simulink model "testing"  (R2020a)
settings: Solver=VariableStepAuto  StartTime=0.0  StopTime=20  RelTol=1e-3
libraries: sps_avr x21, powerlib x17, powerlib_meascontrol x6, spsDieselMotorModel x3
settings Model: Creator=assem  LastModifiedBy=assem

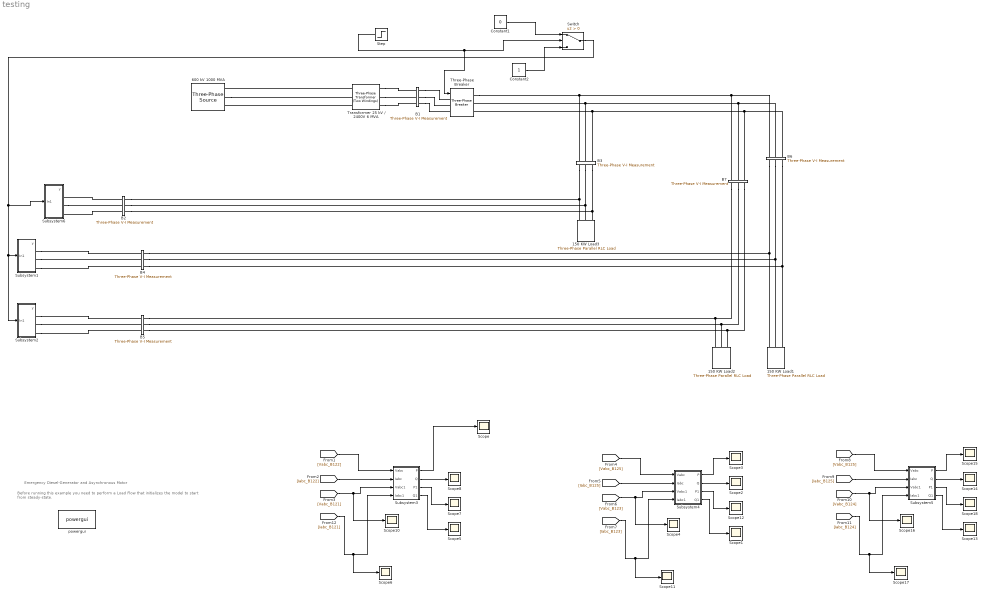
== system testing ==
  note: Emergency Diesel-Generator and Asynchronous Motor
  note: Before running this example you need to perform a Load Flow that
      | initializes the model to start from steady-state.
  150 KW Load1 : powerlib/Elements/Three-Phase Parallel RLC Load  LConnTagsString=A|B|C  Configuration=Y (grounded)  NominalVoltage=2400  Vabc=[1e3 1e3 1e3]  Vabcp=[1e3 1e3 1e3]  NominalFrequency=60  UnbalancedPower=off  ActivePower=.15e+006  InductivePower=0  CapacitivePower=0  Pabc=[10e3 9e3 11e3]  QLabc=[100 90 110]  QCabc=[100 90 110]  Pabcp=[10e3 9e3 11e3]  QLabcp=[100 90 110]  QCabcp=[100 90 110]  Measurements=None  LoadType=constant Z
      settings: SourceProductBaseCode=MT,PS
  150 KW Load2 : powerlib/Elements/Three-Phase Parallel RLC Load  LConnTagsString=A|B|C  Configuration=Y (grounded)  NominalVoltage=2400  Vabc=[1e3 1e3 1e3]  Vabcp=[1e3 1e3 1e3]  NominalFrequency=60  UnbalancedPower=off  ActivePower=.15e+006  InductivePower=0  CapacitivePower=0  Pabc=[10e3 9e3 11e3]  QLabc=[100 90 110]  QCabc=[100 90 110]  Pabcp=[10e3 9e3 11e3]  QLabcp=[100 90 110]  QCabcp=[100 90 110]  Measurements=None  LoadType=constant Z
      settings: SourceProductBaseCode=MT,PS
  150 KW Load3 : powerlib/Elements/Three-Phase Parallel RLC Load  LConnTagsString=A|B|C  Configuration=Y (grounded)  NominalVoltage=2400  Vabc=[1e3 1e3 1e3]  Vabcp=[1e3 1e3 1e3]  NominalFrequency=60  UnbalancedPower=off  ActivePower=.2e+006  InductivePower=0  CapacitivePower=0  Pabc=[10e3 9e3 11e3]  QLabc=[100 90 110]  QCabc=[100 90 110]  Pabcp=[10e3 9e3 11e3]  QLabcp=[100 90 110]  QCabcp=[100 90 110]  Measurements=None  LoadType=constant Z
      settings: SourceProductBaseCode=MT,PS
  600 kV 1000 MVA : powerlib/Electrical Sources/Three-Phase Source  InternalConnection=Yg  VoltagePhases=off  Voltage=(13800)*1  PhaseAngle=0.071468  Voltage_phases=[25e3 25e3 25e3]/sqrt(3)  PhaseAngles_phases=[0 -120 +120]  Frequency=60  NonIdealSource=on  SpecifyImpedance=on  Resistance=25^2/1000/10  Inductance=25^2/1000/377  ShortCircuitLevel=1000e6  BaseVoltage=13.8e3  XRratio=7  BusType=swing  Pref=0  Qref=0  Prefabc=[10e3, 10e3, 10e3]  Qrefabc=[0, 0, 0]  Qmin=-Inf  Qmax=Inf
      settings: SourceProductBaseCode=MT,PS
  B1 : powerlib/Measurements/Three-Phase V-I Measurement  VoltageMeasurement=phase-to-ground  SetLabelV=on  LabelV=Vabc_B120  Vpu=off  VpuLL=off  CurrentMeasurement=yes  SetLabelI=on  LabelI=Iabc_B120  Ipu=off  Pbase=100e6  Vbase=120e3  OutputType=Complex  PhasorSimulation=on  PSBequivalent=0
      settings: SourceProductBaseCode=MT,PS
  B2 : powerlib/Measurements/Three-Phase V-I Measurement  VoltageMeasurement=phase-to-ground  SetLabelV=on  LabelV=Vabc_B121  Vpu=off  VpuLL=off  CurrentMeasurement=yes  SetLabelI=on  LabelI=Iabc_B121  Ipu=off  Pbase=100e6  Vbase=120e3  OutputType=Complex  PhasorSimulation=on  PSBequivalent=0
      settings: SourceProductBaseCode=MT,PS
  B3 : powerlib/Measurements/Three-Phase V-I Measurement  VoltageMeasurement=phase-to-ground  SetLabelV=on  LabelV=Vabc_B122  Vpu=off  VpuLL=off  CurrentMeasurement=yes  SetLabelI=on  LabelI=Iabc_B122  Ipu=off  Pbase=100e6  Vbase=120e3  OutputType=Complex  PhasorSimulation=on  PSBequivalent=0
      settings: SourceProductBaseCode=MT,PS
  B4 : powerlib/Measurements/Three-Phase V-I Measurement  VoltageMeasurement=phase-to-ground  SetLabelV=on  LabelV=Vabc_B123  Vpu=off  VpuLL=off  CurrentMeasurement=yes  SetLabelI=on  LabelI=Iabc_B123  Ipu=off  Pbase=100e6  Vbase=120e3  OutputType=Complex  PhasorSimulation=on  PSBequivalent=0
      settings: SourceProductBaseCode=MT,PS
  B5 : powerlib/Measurements/Three-Phase V-I Measurement  VoltageMeasurement=phase-to-ground  SetLabelV=on  LabelV=Vabc_B124  Vpu=off  VpuLL=off  CurrentMeasurement=yes  SetLabelI=on  LabelI=Iabc_B124  Ipu=off  Pbase=100e6  Vbase=120e3  OutputType=Complex  PhasorSimulation=on  PSBequivalent=0
      settings: SourceProductBaseCode=MT,PS
  B6 : powerlib/Measurements/Three-Phase V-I Measurement  VoltageMeasurement=phase-to-ground  SetLabelV=on  LabelV=Vabc_B125  Vpu=off  VpuLL=off  CurrentMeasurement=yes  SetLabelI=on  LabelI=Iabc_B125  Ipu=off  Pbase=100e6  Vbase=120e3  OutputType=Complex  PhasorSimulation=on  PSBequivalent=0
      settings: SourceProductBaseCode=MT,PS
  B7 : powerlib/Measurements/Three-Phase V-I Measurement  VoltageMeasurement=phase-to-ground  SetLabelV=on  LabelV=Vabc_B126  Vpu=off  VpuLL=off  CurrentMeasurement=yes  SetLabelI=on  LabelI=Iabc_B126  Ipu=off  Pbase=100e6  Vbase=120e3  OutputType=Complex  PhasorSimulation=on  PSBequivalent=0
      settings: SourceProductBaseCode=MT,PS
  Constant1 : Constant  Value=0  SampleTime=1
  Constant2 : Constant  SampleTime=1
  Scope{,1..8,10..18} (18 alike) : Scope
  Step : Step  Time=4  Before=1  After=0  SampleTime=0
  Subsystem1 : Subsystem
  Subsystem2 : Subsystem
  Subsystem3 : Subsystem
  Subsystem4 : Subsystem
  Subsystem5 : Subsystem
  Subsystem6 : Subsystem
  Switch : Switch  Criteria=u2 > Threshold
  Three-Phase Breaker : powerlib/Elements/Three-Phase Breaker  InitialState=closed  SwitchA=on  SwitchB=on  SwitchC=on  SwitchTimes="[1/60  5/60]"  External=on  BreakerResistance=0.01  SnubberResistance=1e6  SnubberCapacitance=inf  Measurements=None
  Transformer 25 kV / 2400V 6 MVA : powerlib/Elements/Three-Phase Transformer (Two Windings)  Winding1Connection=Yg  Winding2Connection=Yg  CoreType=Three single-phase transformers  SetSaturation=off  Hysteresis=off  DataFile='hysteresis'  SetInitialFlux=off  Measurements=None  UNITS=pu  NominalPower=[ 5e6 , 60 ]  Winding1=[13.8e3 0.0015 0.03]  Winding2=[2.4e3 0.0015 0.03]  Rm=200  Lm=200  L0=3.7357e-08  Saturation=[0 0;0.005 1.2;1 1.4]  InitialFluxes=[0.022525 -0.022525 0.019709]  BreakLoop=off  DiscreteSolver=Trapezoidal iterative  DataType=off  TransfoNumber=0
      settings: SourceProductBaseCode=MT,PS
  powergui : powerlib/powergui  Priority=2  SimulationMode=Continuous  SampleTime=50e-6  frequency=60  Iterations=50  frequencyindice=60  Pbase=1e6  ErrMax=0.0001  UnitsV=kV  UnitsW=MW  buscounter=0  FunctionMessages=off  echomessages=off  EnableUseOfTLC=off  CurrentSourceSwitches=off  DisableSnubberDevices=on  DisableRonSwitches=off  DisableVfSwitches=off  DisplayEquations=off  AutomaticDiscreteSolvers=off  SolverType=Tustin  Interpol=off  ExternalGateDelay=off  methode=off  Ts=0  x0status=blocks  SPID=on  SwTol=0  HookPort=off  NonlinearTolerance=1e-4  nMaxIteration=100  ContinueOnMaxIteration=off  RestoreLinks=warning  ResistiveCurrentMeasurement=off  Frange=logspace(0,3,50)  Ylog=off  Xlog=off  ShowGrid=off  save=off  variable=ZData  structure=0  ZoomFFT=on  StartTime=0.0  cycles=2  DisplayStyle=off  fundamental=60  FreqAxis=off  MaxFrequency=1000  frequencyindicesteady=1  RmsSteady=1  display=off
  wires:
  Step/1 -> Three-Phase Breaker/1, Switch/2
  Constant2/1 -> Switch/3
  Constant1/1 -> Switch/1
  Switch/1 -> Subsystem6/1(In1), Subsystem2/1(In1), Subsystem1/1(In1)
  [Vabc_B123] -> Subsystem4/3(Vabc1), Scope4/1
  [Iabc_B123] -> Subsystem4/4(Iabc1), Scope11/1
  Subsystem4/4(Q1) -> Scope1/1
  Subsystem4/1(P) -> Scope3/1
  [Vabc_B125] -> Subsystem4/1(Vabc)
  [Iabc_B125] -> Subsystem4/2(Iabc)
  Subsystem4/2(Q) -> Scope2/1
  Subsystem4/3(P1) -> Scope12/1
  [Vabc_B124] -> Subsystem5/3(Vabc1), Scope16/1
  [Iabc_B124] -> Subsystem5/4(Iabc1), Scope17/1
  Subsystem5/4(Q1) -> Scope13/1
  Subsystem5/1(P) -> Scope15/1
  [Vabc_B125] -> Subsystem5/1(Vabc)
  [Iabc_B125] -> Subsystem5/2(Iabc)
  Subsystem5/2(Q) -> Scope14/1
  Subsystem5/3(P1) -> Scope18/1
  Subsystem3/2(Q) -> Scope8/1
  Subsystem3/3(P1) -> Scope7/1
  [Iabc_B122] -> Subsystem3/2(Iabc)
  [Vabc_B122] -> Subsystem3/1(Vabc)
  [Iabc_B121] -> Subsystem3/4(Iabc1), Scope6/1
  [Vabc_B121] -> Subsystem3/3(Vabc1), Scope10/1
  Subsystem3/4(Q1) -> Scope5/1
  Subsystem3/1(P) -> Scope/1
  connections:
  B1/RConn3 -- Three-Phase Breaker/LConn3
  600 kV 1000 MVA/RConn2 -- Transformer 25 kV / 2400V 6 MVA/LConn2
  Transformer 25 kV / 2400V 6 MVA/RConn1 -- B1/LConn1
  Three-Phase Breaker/RConn1 -- B3/LConn3 -- B7/LConn3 -- B6/RConn3
  B1/RConn2 -- Three-Phase Breaker/LConn2
  Transformer 25 kV / 2400V 6 MVA/RConn2 -- B1/LConn2
  B1/RConn1 -- Three-Phase Breaker/LConn1
  Transformer 25 kV / 2400V 6 MVA/LConn3 -- 600 kV 1000 MVA/RConn3
  Transformer 25 kV / 2400V 6 MVA/LConn1 -- 600 kV 1000 MVA/RConn1
  B6/RConn1 -- B3/LConn1 -- Three-Phase Breaker/RConn3 -- B7/LConn1
  Transformer 25 kV / 2400V 6 MVA/RConn3 -- B1/LConn3
  B6/RConn2 -- B3/LConn2 -- Three-Phase Breaker/RConn2 -- B7/LConn2
  Subsystem1/RConn1 -- B4/LConn1
  Subsystem1/RConn2 -- B4/LConn2
  Subsystem1/RConn3 -- B4/LConn3
  Subsystem2/RConn1 -- B5/LConn1
  Subsystem2/RConn2 -- B5/LConn2
  Subsystem2/RConn3 -- B5/LConn3
  B4/RConn3 -- B6/LConn1 -- 150 KW Load1/LConn3
  B4/RConn2 -- B6/LConn2 -- 150 KW Load1/LConn2
  B4/RConn1 -- B6/LConn3 -- 150 KW Load1/LConn1
  B5/RConn3 -- B7/RConn1 -- 150 KW Load2/LConn3
  B5/RConn2 -- B7/RConn2 -- 150 KW Load2/LConn2
  B5/RConn1 -- B7/RConn3 -- 150 KW Load2/LConn1
  B2/LConn1 -- Subsystem6/RConn1
  Subsystem6/RConn2 -- B2/LConn2
  B2/LConn3 -- Subsystem6/RConn3
  B3/RConn1 -- B2/RConn3 -- 150 KW Load3/LConn3
  B3/RConn2 -- B2/RConn2 -- 150 KW Load3/LConn2
  B3/RConn3 -- B2/RConn1 -- 150 KW Load3/LConn1

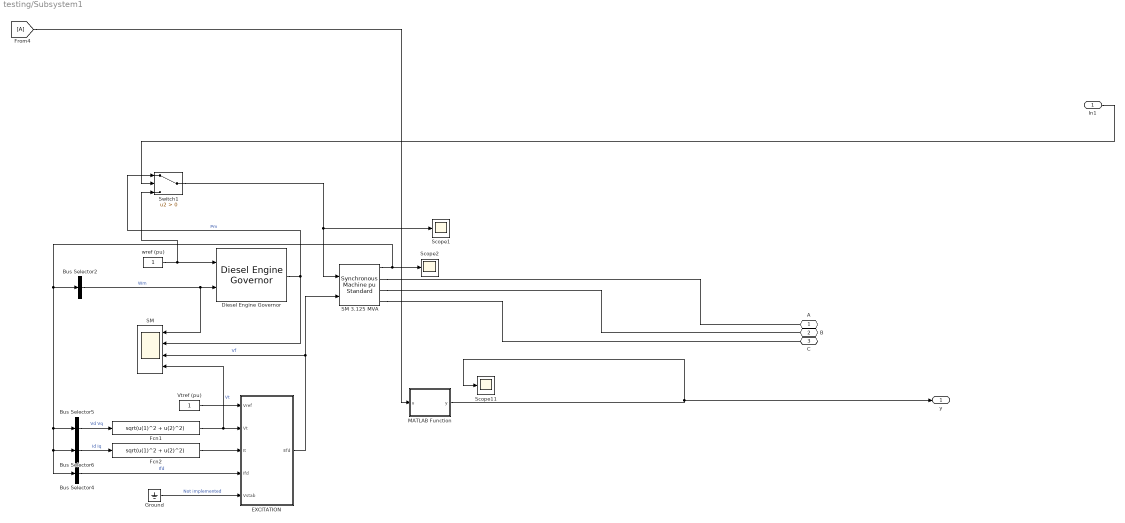
== system testing/Subsystem1 ==
  In1 : Inport
  Bus Selector2 : BusSelector  OutputSignals="Mechanical.Rotor speed  wm  (pu)"  OutputAsBus=on
  Bus Selector4 : BusSelector  OutputSignals="dq0 components.Field current  ifd (pu)"  OutputAsBus=on
  Bus Selector5 : BusSelector  OutputSignals="dq0 components.Stator voltage  vd (pu),dq0 components.Stator voltage  vq (pu)"  OutputAsBus=on
  Bus Selector6 : BusSelector  OutputSignals="dq0 components.Stator current  id (pu),dq0 components.Stator current  iq (pu)"  OutputAsBus=on
  Diesel Engine Governor : spsDieselMotorModel/Diesel Engine Governor  K=40  Tr=[0.01 0.02 0.2]  Ta=[0.25 0.009 0.0384]  Tlim=[0 1.1]  Td=0.024  Pm0=0
      settings: SourceProductBaseCode=MT,PS
  EXCITATION : Subsystem  Variant=on  VariantControlMode=Label  LabelModeActiveChoice=Variant1
      settings: AttributesFormatString=%<BlockChoice>
  Fcn1 : Fcn  Expr=sqrt(u(1)^2 + u(2)^2)
  Fcn2 : Fcn  Expr=sqrt(u(1)^2 + u(2)^2)
  Ground : Ground
  MATLAB Function : MATLAB Function  TreatAsAtomicUnit=on
  SM : Scope  NumInputPorts=4
  SM 3.125 MVA : powerlib/Machines/Synchronous Machine pu Standard  PresetModel=No  MechanicalLoad=Mechanical power Pm  ShowDetailedParameters=on  RotorType=Salient-pole  Units=per unit standard parameters  MeasurementBus=off  NominalParameters="[ .7e6  2400  60]"  Reactances1=[ 31 32 33 34 35 36 37 ]  Reactances2=[ 1.56, 0.296, 0.177, 1.06, 0.177, 0.052 ]  dAxisTimeConstants=Short-circuit  qAxisTimeConstants=Open-circuit  TimeConstants1=[]  TimeConstants2=[]  TimeConstants3=[]  TimeConstants4=[]  TimeConstants5=[ 3.7, 0.05, 0.05 ]  TimeConstants6=[ 8.0, 0.03, 0.3371, 0.0295 ]  TimeConstants7=[0.024 0.006 0.006]  TimeConstants8=[]  StatorResistance=0.0036  Mechanical="[ 1.07  0 2]"  PolePairs=2  InitialConditions=[0 0 0 0 0 0 0 0 1]  SetSaturation=off  Saturation=[0.211 0.418 1.0 1.25 1.72 3.35 ;0.25 0.50 1.0 1.1 1.2 1.4]  LoadFlowParameters=[1 0 0 0]  TsPowergui=0  TsBlock=-1  IterativeModel=Trapezoidal non iterative  IterativeDiscreteModel=Trapezoidal non iterative  BusType=swing  Pref=0  Qref=0  Qmin=-Inf  Qmax=Inf  PLF=0  QLF=0
      settings: AttributesFormatString=\n\n  SourceProductBaseCode=MT,PS
  Scope1 : Scope
  Scope11 : Scope
  Scope2 : Scope
  Switch1 : Switch  Criteria=u2 > Threshold
  "Vtref (pu) " : Constant
  wref (pu) : Constant
  A : PMIOPort  Side=Right
  B : PMIOPort  Port=2  Side=Right
  C : PMIOPort  Port=3  Side=Right
  y : Outport
  wires:
  Switch1/1 -> SM 3.125 MVA/1, Scope1/1
  In1/1 -> Switch1/2
  EXCITATION/1(Efd) -> SM/3, SM 3.125 MVA/2  "Vf"
  wref (pu)/1 -> Switch1/3, Diesel Engine Governor/1
  Bus Selector2/1 -> Diesel Engine Governor/2, SM/1  "Wm"
  "Vtref (pu) "/1 -> EXCITATION/1(Vref)
  Ground/1 -> EXCITATION/5(Vstab)  "Not implemented"
  Fcn2/1 -> EXCITATION/3(It)
  [A] -> MATLAB Function/1(u)
  SM 3.125 MVA/1 -> Bus Selector2/1, Bus Selector5/1, Bus Selector6/1, Bus Selector4/1, Scope2/1
  Bus Selector5/1 -> Fcn1/1  "Vd Vq"
  Fcn1/1 -> SM/4, EXCITATION/2(Vt)  "Vt"
  Bus Selector6/1 -> Fcn2/1  "Id Iq"
  Diesel Engine Governor/1 -> Switch1/1, SM/2  "Pm"
  Bus Selector4/1 -> EXCITATION/4(Ifd)  "Ifd"
  MATLAB Function/1(y) -> y/1, Scope11/1
  connections:
  SM 3.125 MVA/RConn3 -- C/RConn1
  SM 3.125 MVA/RConn1 -- A/RConn1
  SM 3.125 MVA/RConn2 -- B/RConn1

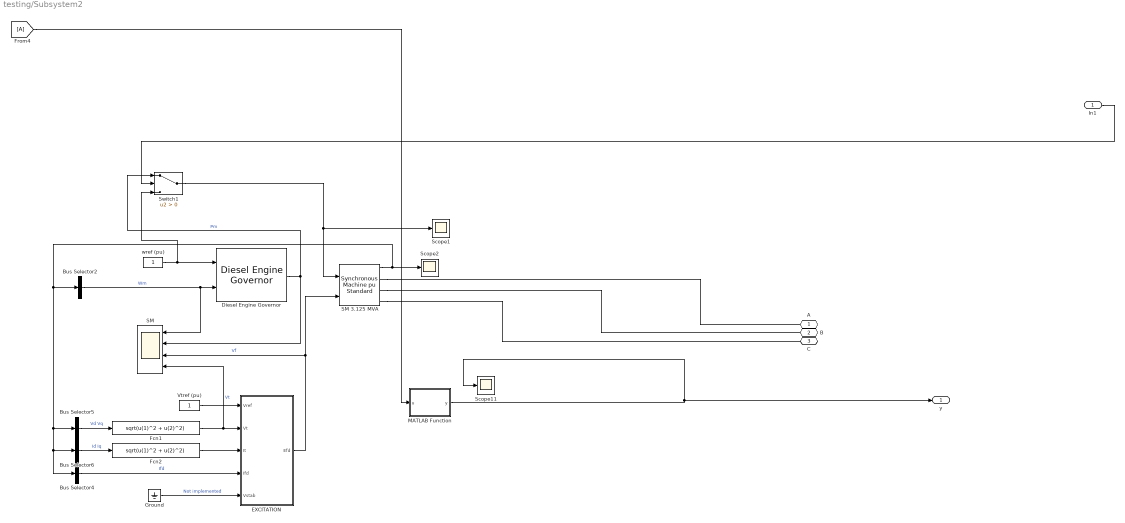
== system testing/Subsystem2 ==
  In1 : Inport
  Bus Selector2 : BusSelector  OutputSignals="Mechanical.Rotor speed  wm  (pu)"  OutputAsBus=on
  Bus Selector4 : BusSelector  OutputSignals="dq0 components.Field current  ifd (pu)"  OutputAsBus=on
  Bus Selector5 : BusSelector  OutputSignals="dq0 components.Stator voltage  vd (pu),dq0 components.Stator voltage  vq (pu)"  OutputAsBus=on
  Bus Selector6 : BusSelector  OutputSignals="dq0 components.Stator current  id (pu),dq0 components.Stator current  iq (pu)"  OutputAsBus=on
  Diesel Engine Governor : spsDieselMotorModel/Diesel Engine Governor  K=40  Tr=[0.01 0.02 0.2]  Ta=[0.25 0.009 0.0384]  Tlim=[0 1.1]  Td=0.024  Pm0=0
      settings: SourceProductBaseCode=MT,PS
  EXCITATION : Subsystem  Variant=on  VariantControlMode=Label  LabelModeActiveChoice=Variant1
      settings: AttributesFormatString=%<BlockChoice>
  Fcn1 : Fcn  Expr=sqrt(u(1)^2 + u(2)^2)
  Fcn2 : Fcn  Expr=sqrt(u(1)^2 + u(2)^2)
  Ground : Ground
  MATLAB Function : MATLAB Function  TreatAsAtomicUnit=on
  SM : Scope  NumInputPorts=4
  SM 3.125 MVA : powerlib/Machines/Synchronous Machine pu Standard  PresetModel=No  MechanicalLoad=Mechanical power Pm  ShowDetailedParameters=on  RotorType=Salient-pole  Units=per unit standard parameters  MeasurementBus=off  NominalParameters="[ .7e6  2400  60]"  Reactances1=[ 31 32 33 34 35 36 37 ]  Reactances2=[ 1.56, 0.296, 0.177, 1.06, 0.177, 0.052 ]  dAxisTimeConstants=Short-circuit  qAxisTimeConstants=Open-circuit  TimeConstants1=[]  TimeConstants2=[]  TimeConstants3=[]  TimeConstants4=[]  TimeConstants5=[ 3.7, 0.05, 0.05 ]  TimeConstants6=[ 8.0, 0.03, 0.3371, 0.0295 ]  TimeConstants7=[0.024 0.006 0.006]  TimeConstants8=[]  StatorResistance=0.0036  Mechanical="[ 1.07  0 2]"  PolePairs=2  InitialConditions=[0 0 0 0 0 0 0 0 1]  SetSaturation=off  Saturation=[0.211 0.418 1.0 1.25 1.72 3.35 ;0.25 0.50 1.0 1.1 1.2 1.4]  LoadFlowParameters=[1 0 0 0]  TsPowergui=0  TsBlock=-1  IterativeModel=Trapezoidal non iterative  IterativeDiscreteModel=Trapezoidal non iterative  BusType=swing  Pref=0  Qref=0  Qmin=-Inf  Qmax=Inf  PLF=0  QLF=0
      settings: AttributesFormatString=\n\n  SourceProductBaseCode=MT,PS
  Scope1 : Scope
  Scope11 : Scope
  Scope2 : Scope
  Switch1 : Switch  Criteria=u2 > Threshold
  "Vtref (pu) " : Constant
  wref (pu) : Constant
  A : PMIOPort  Side=Right
  B : PMIOPort  Port=2  Side=Right
  C : PMIOPort  Port=3  Side=Right
  y : Outport
  wires:
  Switch1/1 -> SM 3.125 MVA/1, Scope1/1
  In1/1 -> Switch1/2
  EXCITATION/1(Efd) -> SM/3, SM 3.125 MVA/2  "Vf"
  wref (pu)/1 -> Switch1/3, Diesel Engine Governor/1
  Bus Selector2/1 -> Diesel Engine Governor/2, SM/1  "Wm"
  "Vtref (pu) "/1 -> EXCITATION/1(Vref)
  Ground/1 -> EXCITATION/5(Vstab)  "Not implemented"
  Fcn2/1 -> EXCITATION/3(It)
  [A] -> MATLAB Function/1(u)
  SM 3.125 MVA/1 -> Bus Selector2/1, Bus Selector5/1, Bus Selector6/1, Bus Selector4/1, Scope2/1
  Bus Selector5/1 -> Fcn1/1  "Vd Vq"
  Fcn1/1 -> SM/4, EXCITATION/2(Vt)  "Vt"
  Bus Selector6/1 -> Fcn2/1  "Id Iq"
  Diesel Engine Governor/1 -> Switch1/1, SM/2  "Pm"
  Bus Selector4/1 -> EXCITATION/4(Ifd)  "Ifd"
  MATLAB Function/1(y) -> y/1, Scope11/1
  connections:
  SM 3.125 MVA/RConn3 -- C/RConn1
  SM 3.125 MVA/RConn1 -- A/RConn1
  SM 3.125 MVA/RConn2 -- B/RConn1

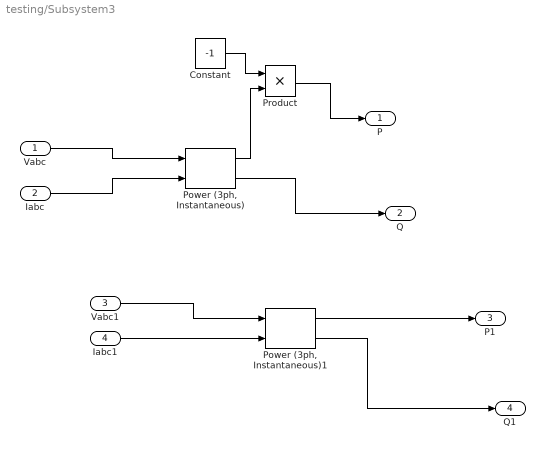
== system testing/Subsystem3 ==
  Vabc : Inport
  Iabc : Inport  Port=2
  Vabc1 : Inport  Port=3
  Iabc1 : Inport  Port=4
  Constant : Constant  Value=-1
  "Power (3ph, Instantaneous)" : powerlib_meascontrol/Measurements/Power (3ph, Instantaneous)
  "Power (3ph, Instantaneous)1" : powerlib_meascontrol/Measurements/Power (3ph, Instantaneous)
  Product : Product
  P : Outport
  Q : Outport  Port=2
  P1 : Outport  Port=3
  Q1 : Outport  Port=4
  wires:
  "Power (3ph, Instantaneous)1"/2 -> Q1/1
  Iabc/1 -> "Power (3ph, Instantaneous)"/2
  "Power (3ph, Instantaneous)1"/1 -> P1/1
  Iabc1/1 -> "Power (3ph, Instantaneous)1"/2
  "Power (3ph, Instantaneous)"/2 -> Q/1
  Vabc1/1 -> "Power (3ph, Instantaneous)1"/1
  Vabc/1 -> "Power (3ph, Instantaneous)"/1
  "Power (3ph, Instantaneous)"/1 -> Product/2
  Constant/1 -> Product/1
  Product/1 -> P/1

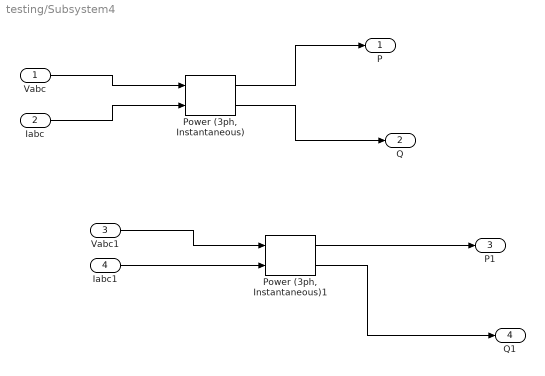
== system testing/Subsystem4 ==
  Vabc : Inport
  Iabc : Inport  Port=2
  Vabc1 : Inport  Port=3
  Iabc1 : Inport  Port=4
  "Power (3ph, Instantaneous)" : powerlib_meascontrol/Measurements/Power (3ph, Instantaneous)
  "Power (3ph, Instantaneous)1" : powerlib_meascontrol/Measurements/Power (3ph, Instantaneous)
  P : Outport
  Q : Outport  Port=2
  P1 : Outport  Port=3
  Q1 : Outport  Port=4
  wires:
  "Power (3ph, Instantaneous)1"/2 -> Q1/1
  "Power (3ph, Instantaneous)"/1 -> P/1
  Iabc/1 -> "Power (3ph, Instantaneous)"/2
  "Power (3ph, Instantaneous)1"/1 -> P1/1
  Iabc1/1 -> "Power (3ph, Instantaneous)1"/2
  "Power (3ph, Instantaneous)"/2 -> Q/1
  Vabc1/1 -> "Power (3ph, Instantaneous)1"/1
  Vabc/1 -> "Power (3ph, Instantaneous)"/1

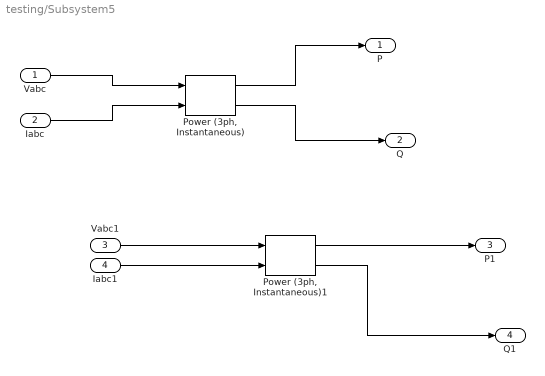
== system testing/Subsystem5 ==
  Vabc : Inport
  Iabc : Inport  Port=2
  Vabc1 : Inport  Port=3
  Iabc1 : Inport  Port=4
  "Power (3ph, Instantaneous)" : powerlib_meascontrol/Measurements/Power (3ph, Instantaneous)
  "Power (3ph, Instantaneous)1" : powerlib_meascontrol/Measurements/Power (3ph, Instantaneous)
  P : Outport
  Q : Outport  Port=2
  P1 : Outport  Port=3
  Q1 : Outport  Port=4
  wires:
  "Power (3ph, Instantaneous)1"/2 -> Q1/1
  "Power (3ph, Instantaneous)"/1 -> P/1
  Iabc/1 -> "Power (3ph, Instantaneous)"/2
  "Power (3ph, Instantaneous)1"/1 -> P1/1
  Iabc1/1 -> "Power (3ph, Instantaneous)1"/2
  "Power (3ph, Instantaneous)"/2 -> Q/1
  Vabc1/1 -> "Power (3ph, Instantaneous)1"/1
  Vabc/1 -> "Power (3ph, Instantaneous)"/1

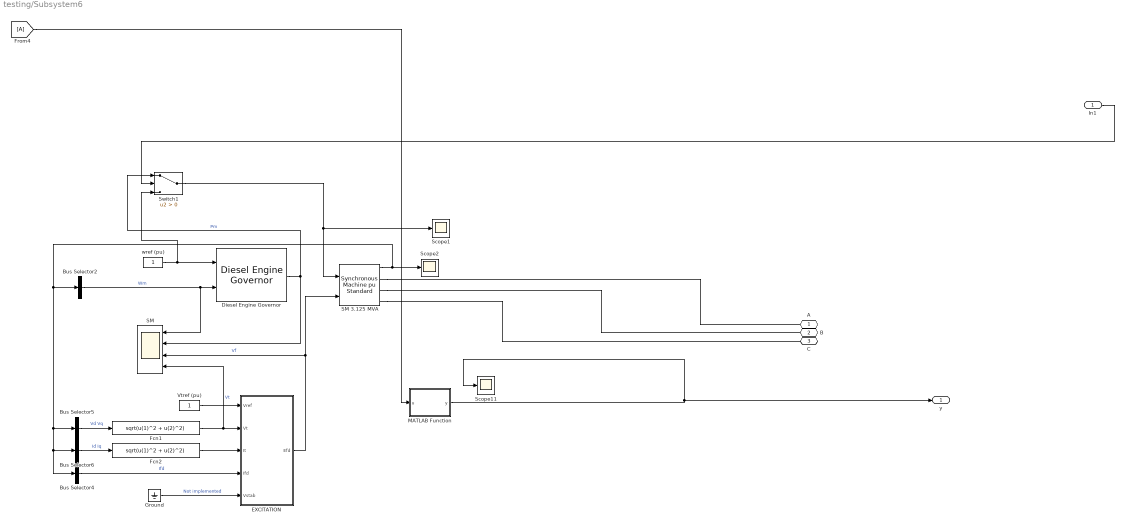
== system testing/Subsystem6 ==
  In1 : Inport
  Bus Selector2 : BusSelector  OutputSignals="Mechanical.Rotor speed  wm  (pu)"  OutputAsBus=on
  Bus Selector4 : BusSelector  OutputSignals="dq0 components.Field current  ifd (pu)"  OutputAsBus=on
  Bus Selector5 : BusSelector  OutputSignals="dq0 components.Stator voltage  vd (pu),dq0 components.Stator voltage  vq (pu)"  OutputAsBus=on
  Bus Selector6 : BusSelector  OutputSignals="dq0 components.Stator current  id (pu),dq0 components.Stator current  iq (pu)"  OutputAsBus=on
  Diesel Engine Governor : spsDieselMotorModel/Diesel Engine Governor  K=40  Tr=[0.01 0.02 0.2]  Ta=[0.25 0.009 0.0384]  Tlim=[0 1.1]  Td=0.024  Pm0=0
      settings: SourceProductBaseCode=MT,PS
  EXCITATION : Subsystem  Variant=on  VariantControlMode=Label  LabelModeActiveChoice=Variant1
      settings: AttributesFormatString=%<BlockChoice>
  Fcn1 : Fcn  Expr=sqrt(u(1)^2 + u(2)^2)
  Fcn2 : Fcn  Expr=sqrt(u(1)^2 + u(2)^2)
  Ground : Ground
  MATLAB Function : MATLAB Function  TreatAsAtomicUnit=on
  SM : Scope  NumInputPorts=4
  SM 3.125 MVA : powerlib/Machines/Synchronous Machine pu Standard  PresetModel=No  MechanicalLoad=Mechanical power Pm  ShowDetailedParameters=on  RotorType=Salient-pole  Units=per unit standard parameters  MeasurementBus=off  NominalParameters="[ .7e6  2400  60]"  Reactances1=[ 31 32 33 34 35 36 37 ]  Reactances2=[ 1.56, 0.296, 0.177, 1.06, 0.177, 0.052 ]  dAxisTimeConstants=Short-circuit  qAxisTimeConstants=Open-circuit  TimeConstants1=[]  TimeConstants2=[]  TimeConstants3=[]  TimeConstants4=[]  TimeConstants5=[ 3.7, 0.05, 0.05 ]  TimeConstants6=[ 8.0, 0.03, 0.3371, 0.0295 ]  TimeConstants7=[0.024 0.006 0.006]  TimeConstants8=[]  StatorResistance=0.0036  Mechanical="[ 1.07  0 2]"  PolePairs=2  InitialConditions=[0 0 0 0 0 0 0 0 1]  SetSaturation=off  Saturation=[0.211 0.418 1.0 1.25 1.72 3.35 ;0.25 0.50 1.0 1.1 1.2 1.4]  LoadFlowParameters=[1 0 0 0]  TsPowergui=0  TsBlock=-1  IterativeModel=Trapezoidal non iterative  IterativeDiscreteModel=Trapezoidal non iterative  BusType=swing  Pref=0  Qref=0  Qmin=-Inf  Qmax=Inf  PLF=0  QLF=0
      settings: AttributesFormatString=\n\n  SourceProductBaseCode=MT,PS
  Scope1 : Scope
  Scope11 : Scope
  Scope2 : Scope
  Switch1 : Switch  Criteria=u2 > Threshold
  "Vtref (pu) " : Constant
  wref (pu) : Constant
  A : PMIOPort  Side=Right
  B : PMIOPort  Port=2  Side=Right
  C : PMIOPort  Port=3  Side=Right
  y : Outport
  wires:
  Switch1/1 -> SM 3.125 MVA/1, Scope1/1
  In1/1 -> Switch1/2
  EXCITATION/1(Efd) -> SM/3, SM 3.125 MVA/2  "Vf"
  wref (pu)/1 -> Switch1/3, Diesel Engine Governor/1
  Bus Selector2/1 -> Diesel Engine Governor/2, SM/1  "Wm"
  "Vtref (pu) "/1 -> EXCITATION/1(Vref)
  Ground/1 -> EXCITATION/5(Vstab)  "Not implemented"
  Fcn2/1 -> EXCITATION/3(It)
  [A] -> MATLAB Function/1(u)
  SM 3.125 MVA/1 -> Bus Selector2/1, Bus Selector5/1, Bus Selector6/1, Bus Selector4/1, Scope2/1
  Bus Selector5/1 -> Fcn1/1  "Vd Vq"
  Fcn1/1 -> SM/4, EXCITATION/2(Vt)  "Vt"
  Bus Selector6/1 -> Fcn2/1  "Id Iq"
  Diesel Engine Governor/1 -> Switch1/1, SM/2  "Pm"
  Bus Selector4/1 -> EXCITATION/4(Ifd)  "Ifd"
  MATLAB Function/1(y) -> y/1, Scope11/1
  connections:
  SM 3.125 MVA/RConn3 -- C/RConn1
  SM 3.125 MVA/RConn1 -- A/RConn1
  SM 3.125 MVA/RConn2 -- B/RConn1

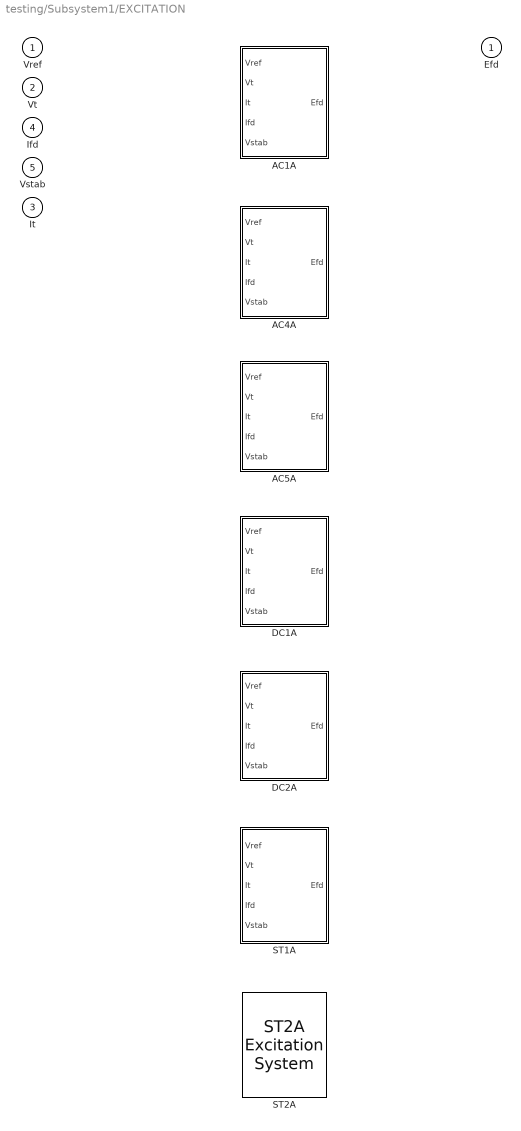
== system testing/Subsystem1/EXCITATION ==
  Vref : Inport
  Vt : Inport  Port=2
  It : Inport  Port=3
  Ifd : Inport  Port=4
  Vstab : Inport  Port=5
  AC1A : Subsystem  VariantControl=Variant1
  AC4A : Subsystem  VariantControl=Variant2
  AC5A : Subsystem  VariantControl=Variant3
  DC1A : Subsystem  VariantControl=Variant4
  DC2A : Subsystem  VariantControl=Variant5
  ST1A : Subsystem  VariantControl=Variant6
  ST2A : sps_avr/ST2A Excitation System  VariantControl=Variant7  Tr=20e-3  KaTa=[120 0.15]  VRminmax=[0 1.0]  KfTf=[0.05 1.0]  KeTe=[1.0 0.5]  KI=8.0  Kp=4.88  Xd=1.56  Kc=1.82  v0=[1,1.42734]  I0=0.2739  TsBlock=-2
      settings: SourceProductBaseCode=MT,PS
  Efd : Outport  VectorParamsAs1DForOutWhenUnconnected=off

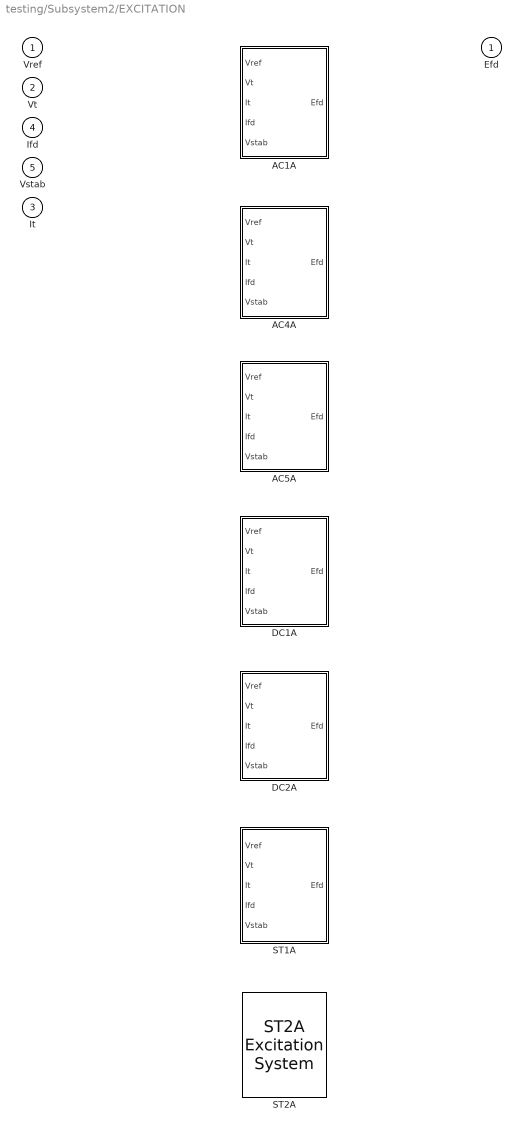
== system testing/Subsystem2/EXCITATION ==
  Vref : Inport
  Vt : Inport  Port=2
  It : Inport  Port=3
  Ifd : Inport  Port=4
  Vstab : Inport  Port=5
  AC1A : Subsystem  VariantControl=Variant1
  AC4A : Subsystem  VariantControl=Variant2
  AC5A : Subsystem  VariantControl=Variant3
  DC1A : Subsystem  VariantControl=Variant4
  DC2A : Subsystem  VariantControl=Variant5
  ST1A : Subsystem  VariantControl=Variant6
  ST2A : sps_avr/ST2A Excitation System  VariantControl=Variant7  Tr=20e-3  KaTa=[120 0.15]  VRminmax=[0 1.0]  KfTf=[0.05 1.0]  KeTe=[1.0 0.5]  KI=8.0  Kp=4.88  Xd=1.56  Kc=1.82  v0=[1,1.42734]  I0=0.2739  TsBlock=-2
      settings: SourceProductBaseCode=MT,PS
  Efd : Outport  VectorParamsAs1DForOutWhenUnconnected=off

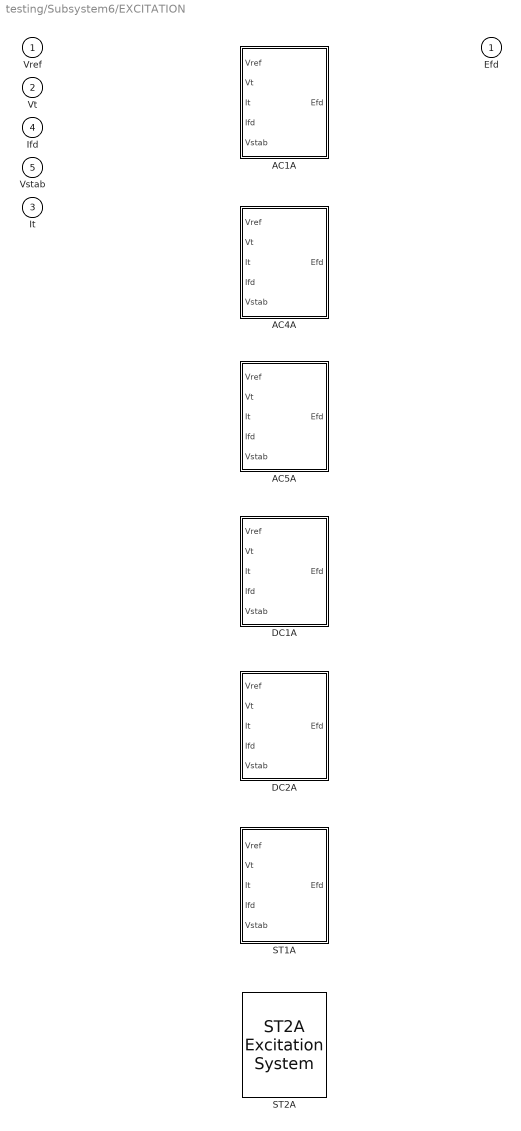
== system testing/Subsystem6/EXCITATION ==
  Vref : Inport
  Vt : Inport  Port=2
  It : Inport  Port=3
  Ifd : Inport  Port=4
  Vstab : Inport  Port=5
  AC1A : Subsystem  VariantControl=Variant1
  AC4A : Subsystem  VariantControl=Variant2
  AC5A : Subsystem  VariantControl=Variant3
  DC1A : Subsystem  VariantControl=Variant4
  DC2A : Subsystem  VariantControl=Variant5
  ST1A : Subsystem  VariantControl=Variant6
  ST2A : sps_avr/ST2A Excitation System  VariantControl=Variant7  Tr=20e-3  KaTa=[120 0.15]  VRminmax=[0 1.0]  KfTf=[0.05 1.0]  KeTe=[1.0 0.5]  KI=8.0  Kp=4.88  Xd=1.56  Kc=1.82  v0=[1,1.42734]  I0=0.2739  TsBlock=-2
      settings: SourceProductBaseCode=MT,PS
  Efd : Outport  VectorParamsAs1DForOutWhenUnconnected=off

== system testing/Subsystem1/EXCITATION/AC1A ==
  Vref : Inport
  Vt : Inport  Port=2
  It : Inport  Port=3
  Ifd : Inport  Port=4
  Vstab : Inport  Port=5
  AC1A : sps_avr/AC1A Excitation System  Tr=20e-3  KaTa=[400 0.02]  VAminmax=[-14.5 14.5]  VRminmax=[-5.43 6.03]  KfTf=[0.03 1.0]  TbTc=[0 0]  KeTe=[1.0 0.80]  Ve12=[4.18 3.14]  SeVe12=[0.10 0.03]  Kd=0.38  Kc=0.20  v0=[1 1.4273]  TsBlock=-2
      settings: SourceProductBaseCode=MT,PS
  term3 : Terminator
  Efd : Outport  VectorParamsAs1DForOutWhenUnconnected=off
  wires:
  It/1 -> term3/1
  AC1A/1 -> Efd/1
  Vstab/1 -> AC1A/4
  Ifd/1 -> AC1A/3
  Vt/1 -> AC1A/2
  Vref/1 -> AC1A/1

== system testing/Subsystem1/EXCITATION/AC4A ==
  Vref : Inport
  Vt : Inport  Port=2
  It : Inport  Port=3
  Ifd : Inport  Port=4
  Vstab : Inport  Port=5
  AC4A : sps_avr/AC4A Excitation System  Tr=20e-3  KaTa=[200 0.015]  VIminmax=[-10 10]  VRminmax=[-4.53 5.64]  TbTc=[10 1.0]  Kc=0  v0=[1,1.42734]  TsBlock=-2
      settings: SourceProductBaseCode=MT,PS
  term3 : Terminator
  Efd : Outport  VectorParamsAs1DForOutWhenUnconnected=off
  wires:
  It/1 -> term3/1
  AC4A/1 -> Efd/1
  Vstab/1 -> AC4A/4
  Ifd/1 -> AC4A/3
  Vt/1 -> AC4A/2
  Vref/1 -> AC4A/1

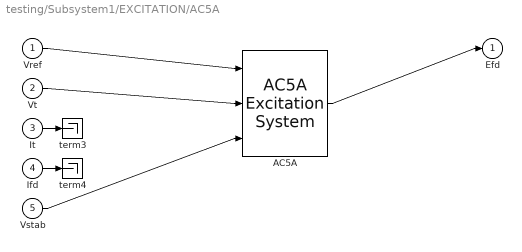
== system testing/Subsystem1/EXCITATION/AC5A ==
  Vref : Inport
  Vt : Inport  Port=2
  It : Inport  Port=3
  Ifd : Inport  Port=4
  Vstab : Inport  Port=5
  AC5A : sps_avr/AC5A Excitation System  Tr=20e-3  KaTa=[100 0.02]  VRminmax=[-7.3 7.3]  KfTf=[0.03 1 0 0]  KeTe=[1.0 0.02]  Efd12=[5.6 0.75*5.6]  SeEfd12=[0.86 0.5]  v0=[1,1.42734]  TsBlock=-2
      settings: SourceProductBaseCode=MT,PS
  term3 : Terminator
  term4 : Terminator
  Efd : Outport  VectorParamsAs1DForOutWhenUnconnected=off
  wires:
  Ifd/1 -> term4/1
  It/1 -> term3/1
  AC5A/1 -> Efd/1
  Vstab/1 -> AC5A/3
  Vt/1 -> AC5A/2
  Vref/1 -> AC5A/1

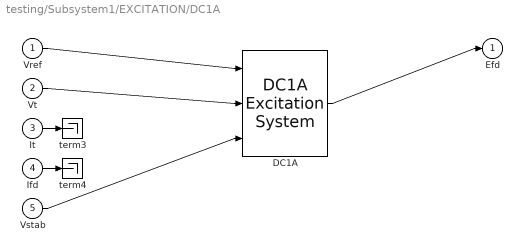
== system testing/Subsystem1/EXCITATION/DC1A ==
  Vref : Inport
  Vt : Inport  Port=2
  It : Inport  Port=3
  Ifd : Inport  Port=4
  Vstab : Inport  Port=5
  DC1A : sps_avr/DC1A Excitation System  Tr=20e-3  KaTa=[46 0.06]  VRminmax=[-0.9 1.0]  KfTf=[0.05 1.5]  TbTc=[0 0]  KeTe=[0.05 0.46]  Efd12=[3.1 2.3]  SeEfd12=[0.33 0.10]  v0=[1,1.42734]  TsBlock=-2
      settings: SourceProductBaseCode=MT,PS
  term3 : Terminator
  term4 : Terminator
  Efd : Outport  VectorParamsAs1DForOutWhenUnconnected=off
  wires:
  Ifd/1 -> term4/1
  It/1 -> term3/1
  DC1A/1 -> Efd/1
  Vstab/1 -> DC1A/3
  Vt/1 -> DC1A/2
  Vref/1 -> DC1A/1

== system testing/Subsystem1/EXCITATION/DC2A ==
  Vref : Inport
  Vt : Inport  Port=2
  It : Inport  Port=3
  Ifd : Inport  Port=4
  Vstab : Inport  Port=5
  DC2A : sps_avr/DC2A Excitation System  Tr=20e-3  KaTa=[46 0.06]  VRminmax=[-4.9 4.95]  KfTf=[0.05 1.5]  TbTc=[0 0]  KeTe=[0.05 0.46]  Efd12=[3.05 2.29]  SeEfd12=[0.279 0.117]  v0=[1,1.42734]  TsBlock=-2
      settings: SourceProductBaseCode=MT,PS
  term3 : Terminator
  term4 : Terminator
  Efd : Outport  VectorParamsAs1DForOutWhenUnconnected=off
  wires:
  Ifd/1 -> term4/1
  It/1 -> term3/1
  DC2A/1 -> Efd/1
  Vstab/1 -> DC2A/3
  Vt/1 -> DC2A/2
  Vref/1 -> DC2A/1

== system testing/Subsystem1/EXCITATION/ST1A ==
  Vref : Inport
  Vt : Inport  Port=2
  It : Inport  Port=3
  Ifd : Inport  Port=4
  Vstab : Inport  Port=5
  ST1A : sps_avr/ST1A Excitation System  Tr=20e-3  KaTa=[210 0.001]  VIminmax=[-999 999]  VAminmax=[-999 999]  VRminmax=[-6.0 6.43]  KfTf=[0.001 1]  TbTc=[0 0 0 0]  KLR=1  ILR=2  Kc=0.038  v0=[1,1.42734]  TsBlock=-2
      settings: SourceProductBaseCode=MT,PS
  term3 : Terminator
  Efd : Outport  VectorParamsAs1DForOutWhenUnconnected=off
  wires:
  It/1 -> term3/1
  ST1A/1 -> Efd/1
  Vstab/1 -> ST1A/4
  Ifd/1 -> ST1A/3
  Vt/1 -> ST1A/2
  Vref/1 -> ST1A/1

== system testing/Subsystem2/EXCITATION/AC1A ==
  Vref : Inport
  Vt : Inport  Port=2
  It : Inport  Port=3
  Ifd : Inport  Port=4
  Vstab : Inport  Port=5
  AC1A : sps_avr/AC1A Excitation System  Tr=20e-3  KaTa=[400 0.02]  VAminmax=[-14.5 14.5]  VRminmax=[-5.43 6.03]  KfTf=[0.03 1.0]  TbTc=[0 0]  KeTe=[1.0 0.80]  Ve12=[4.18 3.14]  SeVe12=[0.10 0.03]  Kd=0.38  Kc=0.20  v0=[1 1.4273]  TsBlock=-2
      settings: SourceProductBaseCode=MT,PS
  term3 : Terminator
  Efd : Outport  VectorParamsAs1DForOutWhenUnconnected=off
  wires:
  It/1 -> term3/1
  AC1A/1 -> Efd/1
  Vstab/1 -> AC1A/4
  Ifd/1 -> AC1A/3
  Vt/1 -> AC1A/2
  Vref/1 -> AC1A/1

== system testing/Subsystem2/EXCITATION/AC4A ==
  Vref : Inport
  Vt : Inport  Port=2
  It : Inport  Port=3
  Ifd : Inport  Port=4
  Vstab : Inport  Port=5
  AC4A : sps_avr/AC4A Excitation System  Tr=20e-3  KaTa=[200 0.015]  VIminmax=[-10 10]  VRminmax=[-4.53 5.64]  TbTc=[10 1.0]  Kc=0  v0=[1,1.42734]  TsBlock=-2
      settings: SourceProductBaseCode=MT,PS
  term3 : Terminator
  Efd : Outport  VectorParamsAs1DForOutWhenUnconnected=off
  wires:
  It/1 -> term3/1
  AC4A/1 -> Efd/1
  Vstab/1 -> AC4A/4
  Ifd/1 -> AC4A/3
  Vt/1 -> AC4A/2
  Vref/1 -> AC4A/1

== system testing/Subsystem2/EXCITATION/AC5A ==
  Vref : Inport
  Vt : Inport  Port=2
  It : Inport  Port=3
  Ifd : Inport  Port=4
  Vstab : Inport  Port=5
  AC5A : sps_avr/AC5A Excitation System  Tr=20e-3  KaTa=[100 0.02]  VRminmax=[-7.3 7.3]  KfTf=[0.03 1 0 0]  KeTe=[1.0 0.02]  Efd12=[5.6 0.75*5.6]  SeEfd12=[0.86 0.5]  v0=[1,1.42734]  TsBlock=-2
      settings: SourceProductBaseCode=MT,PS
  term3 : Terminator
  term4 : Terminator
  Efd : Outport  VectorParamsAs1DForOutWhenUnconnected=off
  wires:
  Ifd/1 -> term4/1
  It/1 -> term3/1
  AC5A/1 -> Efd/1
  Vstab/1 -> AC5A/3
  Vt/1 -> AC5A/2
  Vref/1 -> AC5A/1

== system testing/Subsystem2/EXCITATION/DC1A ==
  Vref : Inport
  Vt : Inport  Port=2
  It : Inport  Port=3
  Ifd : Inport  Port=4
  Vstab : Inport  Port=5
  DC1A : sps_avr/DC1A Excitation System  Tr=20e-3  KaTa=[46 0.06]  VRminmax=[-0.9 1.0]  KfTf=[0.05 1.5]  TbTc=[0 0]  KeTe=[0.05 0.46]  Efd12=[3.1 2.3]  SeEfd12=[0.33 0.10]  v0=[1,1.42734]  TsBlock=-2
      settings: SourceProductBaseCode=MT,PS
  term3 : Terminator
  term4 : Terminator
  Efd : Outport  VectorParamsAs1DForOutWhenUnconnected=off
  wires:
  Ifd/1 -> term4/1
  It/1 -> term3/1
  DC1A/1 -> Efd/1
  Vstab/1 -> DC1A/3
  Vt/1 -> DC1A/2
  Vref/1 -> DC1A/1

== system testing/Subsystem2/EXCITATION/DC2A ==
  Vref : Inport
  Vt : Inport  Port=2
  It : Inport  Port=3
  Ifd : Inport  Port=4
  Vstab : Inport  Port=5
  DC2A : sps_avr/DC2A Excitation System  Tr=20e-3  KaTa=[46 0.06]  VRminmax=[-4.9 4.95]  KfTf=[0.05 1.5]  TbTc=[0 0]  KeTe=[0.05 0.46]  Efd12=[3.05 2.29]  SeEfd12=[0.279 0.117]  v0=[1,1.42734]  TsBlock=-2
      settings: SourceProductBaseCode=MT,PS
  term3 : Terminator
  term4 : Terminator
  Efd : Outport  VectorParamsAs1DForOutWhenUnconnected=off
  wires:
  Ifd/1 -> term4/1
  It/1 -> term3/1
  DC2A/1 -> Efd/1
  Vstab/1 -> DC2A/3
  Vt/1 -> DC2A/2
  Vref/1 -> DC2A/1

== system testing/Subsystem2/EXCITATION/ST1A ==
  Vref : Inport
  Vt : Inport  Port=2
  It : Inport  Port=3
  Ifd : Inport  Port=4
  Vstab : Inport  Port=5
  ST1A : sps_avr/ST1A Excitation System  Tr=20e-3  KaTa=[210 0.001]  VIminmax=[-999 999]  VAminmax=[-999 999]  VRminmax=[-6.0 6.43]  KfTf=[0.001 1]  TbTc=[0 0 0 0]  KLR=1  ILR=2  Kc=0.038  v0=[1,1.42734]  TsBlock=-2
      settings: SourceProductBaseCode=MT,PS
  term3 : Terminator
  Efd : Outport  VectorParamsAs1DForOutWhenUnconnected=off
  wires:
  It/1 -> term3/1
  ST1A/1 -> Efd/1
  Vstab/1 -> ST1A/4
  Ifd/1 -> ST1A/3
  Vt/1 -> ST1A/2
  Vref/1 -> ST1A/1

== system testing/Subsystem6/EXCITATION/AC1A ==
  Vref : Inport
  Vt : Inport  Port=2
  It : Inport  Port=3
  Ifd : Inport  Port=4
  Vstab : Inport  Port=5
  AC1A : sps_avr/AC1A Excitation System  Tr=20e-3  KaTa=[400 0.02]  VAminmax=[-14.5 14.5]  VRminmax=[-5.43 6.03]  KfTf=[0.03 1.0]  TbTc=[0 0]  KeTe=[1.0 0.80]  Ve12=[4.18 3.14]  SeVe12=[0.10 0.03]  Kd=0.38  Kc=0.20  v0=[1 1.4273]  TsBlock=-2
      settings: SourceProductBaseCode=MT,PS
  term3 : Terminator
  Efd : Outport  VectorParamsAs1DForOutWhenUnconnected=off
  wires:
  It/1 -> term3/1
  AC1A/1 -> Efd/1
  Vstab/1 -> AC1A/4
  Ifd/1 -> AC1A/3
  Vt/1 -> AC1A/2
  Vref/1 -> AC1A/1

== system testing/Subsystem6/EXCITATION/AC4A ==
  Vref : Inport
  Vt : Inport  Port=2
  It : Inport  Port=3
  Ifd : Inport  Port=4
  Vstab : Inport  Port=5
  AC4A : sps_avr/AC4A Excitation System  Tr=20e-3  KaTa=[200 0.015]  VIminmax=[-10 10]  VRminmax=[-4.53 5.64]  TbTc=[10 1.0]  Kc=0  v0=[1,1.42734]  TsBlock=-2
      settings: SourceProductBaseCode=MT,PS
  term3 : Terminator
  Efd : Outport  VectorParamsAs1DForOutWhenUnconnected=off
  wires:
  It/1 -> term3/1
  AC4A/1 -> Efd/1
  Vstab/1 -> AC4A/4
  Ifd/1 -> AC4A/3
  Vt/1 -> AC4A/2
  Vref/1 -> AC4A/1

== system testing/Subsystem6/EXCITATION/AC5A ==
  Vref : Inport
  Vt : Inport  Port=2
  It : Inport  Port=3
  Ifd : Inport  Port=4
  Vstab : Inport  Port=5
  AC5A : sps_avr/AC5A Excitation System  Tr=20e-3  KaTa=[100 0.02]  VRminmax=[-7.3 7.3]  KfTf=[0.03 1 0 0]  KeTe=[1.0 0.02]  Efd12=[5.6 0.75*5.6]  SeEfd12=[0.86 0.5]  v0=[1,1.42734]  TsBlock=-2
      settings: SourceProductBaseCode=MT,PS
  term3 : Terminator
  term4 : Terminator
  Efd : Outport  VectorParamsAs1DForOutWhenUnconnected=off
  wires:
  Ifd/1 -> term4/1
  It/1 -> term3/1
  AC5A/1 -> Efd/1
  Vstab/1 -> AC5A/3
  Vt/1 -> AC5A/2
  Vref/1 -> AC5A/1

== system testing/Subsystem6/EXCITATION/DC1A ==
  Vref : Inport
  Vt : Inport  Port=2
  It : Inport  Port=3
  Ifd : Inport  Port=4
  Vstab : Inport  Port=5
  DC1A : sps_avr/DC1A Excitation System  Tr=20e-3  KaTa=[46 0.06]  VRminmax=[-0.9 1.0]  KfTf=[0.05 1.5]  TbTc=[0 0]  KeTe=[0.05 0.46]  Efd12=[3.1 2.3]  SeEfd12=[0.33 0.10]  v0=[1,1.42734]  TsBlock=-2
      settings: SourceProductBaseCode=MT,PS
  term3 : Terminator
  term4 : Terminator
  Efd : Outport  VectorParamsAs1DForOutWhenUnconnected=off
  wires:
  Ifd/1 -> term4/1
  It/1 -> term3/1
  DC1A/1 -> Efd/1
  Vstab/1 -> DC1A/3
  Vt/1 -> DC1A/2
  Vref/1 -> DC1A/1

== system testing/Subsystem6/EXCITATION/DC2A ==
  Vref : Inport
  Vt : Inport  Port=2
  It : Inport  Port=3
  Ifd : Inport  Port=4
  Vstab : Inport  Port=5
  DC2A : sps_avr/DC2A Excitation System  Tr=20e-3  KaTa=[46 0.06]  VRminmax=[-4.9 4.95]  KfTf=[0.05 1.5]  TbTc=[0 0]  KeTe=[0.05 0.46]  Efd12=[3.05 2.29]  SeEfd12=[0.279 0.117]  v0=[1,1.42734]  TsBlock=-2
      settings: SourceProductBaseCode=MT,PS
  term3 : Terminator
  term4 : Terminator
  Efd : Outport  VectorParamsAs1DForOutWhenUnconnected=off
  wires:
  Ifd/1 -> term4/1
  It/1 -> term3/1
  DC2A/1 -> Efd/1
  Vstab/1 -> DC2A/3
  Vt/1 -> DC2A/2
  Vref/1 -> DC2A/1

== system testing/Subsystem6/EXCITATION/ST1A ==
  Vref : Inport
  Vt : Inport  Port=2
  It : Inport  Port=3
  Ifd : Inport  Port=4
  Vstab : Inport  Port=5
  ST1A : sps_avr/ST1A Excitation System  Tr=20e-3  KaTa=[210 0.001]  VIminmax=[-999 999]  VAminmax=[-999 999]  VRminmax=[-6.0 6.43]  KfTf=[0.001 1]  TbTc=[0 0 0 0]  KLR=1  ILR=2  Kc=0.038  v0=[1,1.42734]  TsBlock=-2
      settings: SourceProductBaseCode=MT,PS
  term3 : Terminator
  Efd : Outport  VectorParamsAs1DForOutWhenUnconnected=off
  wires:
  It/1 -> term3/1
  ST1A/1 -> Efd/1
  Vstab/1 -> ST1A/4
  Ifd/1 -> ST1A/3
  Vt/1 -> ST1A/2
  Vref/1 -> ST1A/1

== matlab function testing/Subsystem6/MATLAB Function ==
  data: u input; y output
function y = fcn(u)
if (u>60.5)
    y=1;
elseif (u<57.5)
   
    y=0;
    
else
    y=1;
end
end

== matlab function testing/Subsystem2/MATLAB Function ==
  data: u input; y output
function y = fcn(u)
if (u>60.5)
    y=1;
elseif (u<57.5)
   
    y=0;
    
else
    y=1;
end
end

== matlab function testing/Subsystem1/MATLAB Function ==
  data: u input; y output
function y = fcn(u)
if (u>60.5)
    y=1;
elseif (u<57.5)
   
    y=0;
    
else
    y=1;
end
end
